simulink model "BlockDiagram"  (R2022a)
settings: Solver=VariableStepAuto  StartTime=0.0  StopTime=10.0  RelTol=1e-3
settings Model: Creator=nikki  LastModifiedBy=nikki

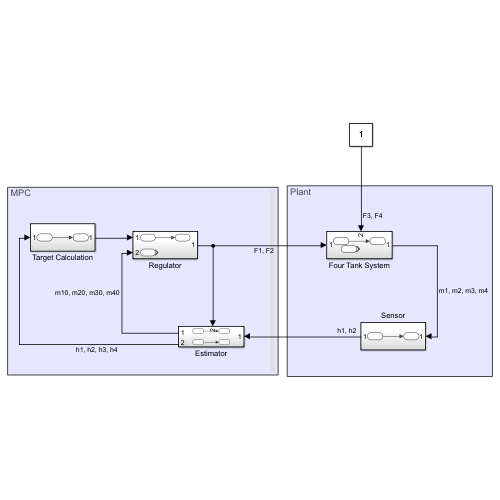
[thumbnail: Simulink's stored preview of the top-level diagram]
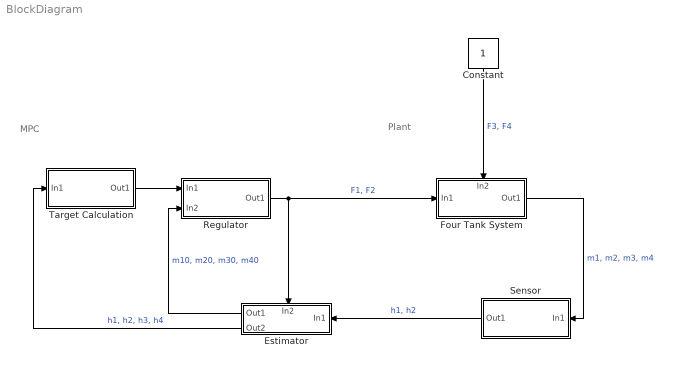
== system BlockDiagram ==
  note: Plant
  note: MPC
  Constant : Constant
  Estimator : Subsystem
      settings: PortSchema="{\"entries\":[{\"content\":{\"sides\":[{\"content\":{\"connectorIds\":[\"In1\"]},\"type\":\"ConnectorPlacement.EquallySpacedRectSide\",\"uuid\":\"54d26656-d64f-4d11-ab89-12a8e0cdd5fe\"},{\"content\":{\"connectorIds\":[\"Out1\",\"Out2\"],\"side\":\"RIGHT\"},\"type\":\"ConnectorPlacement.EquallySpacedRectSide\",\"uuid\":\"a230d698-0203-466e-ba98-0369b8efe661\"},{\"content\":{\"connectorIds\":[\"In2\"],\"side\":\"TOP\"},\"type\":\"ConnectorPlacement.EquallySpacedRectSide\",\"uuid\":\"06e4e78b-3cb8-45b8-ad05-1124743348f7\"},{\"content\":{\"connectorIds\":[],\"side\":\"BOTTOM\"},\"type\":\"ConnectorPlacement.EquallySpacedRectSide\",\"uuid\":\"bba1e365-74c6-4fbc-b191-71d86407624c\"}]},\"type\":\"ConnectorPlacement.EquallySpacedConnector\",\"uuid\":\"ea5774ef-2a07-4a32-9146-0fb2b6d861d1\"}],\"packageUris\":[\"http://schema.mathworks.com/mf0/Connector/R2020b\"],\"version\":\"1.0\"}"
  Four Tank System : Subsystem
      settings: PortSchema="{\"entries\":[{\"content\":{\"sides\":[{\"content\":{\"connectorIds\":[\"In1\"]},\"type\":\"ConnectorPlacement.EquallySpacedRectSide\",\"uuid\":\"54d26656-d64f-4d11-ab89-12a8e0cdd5fe\"},{\"content\":{\"connectorIds\":[\"Out1\"],\"side\":\"RIGHT\"},\"type\":\"ConnectorPlacement.EquallySpacedRectSide\",\"uuid\":\"a230d698-0203-466e-ba98-0369b8efe661\"},{\"content\":{\"connectorIds\":[\"In2\"],\"side\":\"TOP\"},\"type\":\"ConnectorPlacement.EquallySpacedRectSide\",\"uuid\":\"06e4e78b-3cb8-45b8-ad05-1124743348f7\"}]},\"type\":\"ConnectorPlacement.EquallySpacedConnector\",\"uuid\":\"ea5774ef-2a07-4a32-9146-0fb2b6d861d1\"}],\"packageUris\":[\"http://schema.mathworks.com/mf0/Connector/R2020b\"],\"version\":\"1.0\"}"
  Regulator : Subsystem
  Sensor : Subsystem
  Target Calculation : Subsystem
  wires:
  Estimator/2(Out2) -> Target Calculation/1(In1)  "h1, h2, h3, h4"
  Estimator/1(Out1) -> Regulator/2(In2)  "m10, m20, m30, m40"
  Target Calculation/1(Out1) -> Regulator/1(In1)
  Regulator/1(Out1) -> Four Tank System/1(In1), Estimator/2(In2)  "F1, F2"
  Constant/1 -> Four Tank System/2(In2)  "F3, F4"
  Sensor/1(Out1) -> Estimator/1(In1)  "h1, h2"
  Four Tank System/1(Out1) -> Sensor/1(In1)  "m1, m2, m3, m4"

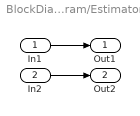
== system BlockDiagram/Estimator ==
  In1 : Inport
  In2 : Inport  Port=2
  Out1 : Outport
  Out2 : Outport  Port=2
  wires:
  In1/1 -> Out1/1
  In2/1 -> Out2/1

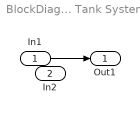
== system BlockDiagram/Four Tank System ==
  In1 : Inport
  In2 : Inport  Port=2
  Out1 : Outport
  wires:
  In1/1 -> Out1/1

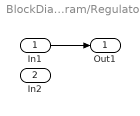
== system BlockDiagram/Regulator ==
  In1 : Inport
  In2 : Inport  Port=2
  Out1 : Outport
  wires:
  In1/1 -> Out1/1

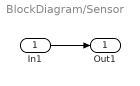
== system BlockDiagram/Sensor ==
  In1 : Inport
  Out1 : Outport
  wires:
  In1/1 -> Out1/1

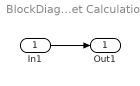
== system BlockDiagram/Target Calculation ==
  In1 : Inport
  Out1 : Outport
  wires:
  In1/1 -> Out1/1
